simulink model "modemPSK"  (Simulink 7.1)
settings: Solver=ode45  StartTime=0.0  StopTime=0.09  RelTol=1e-3
libraries: dsparch4 x2, simulink x1, commrandsrc2 x1
settings Model: Creator=David Castro  LastModifiedBy=David Castro

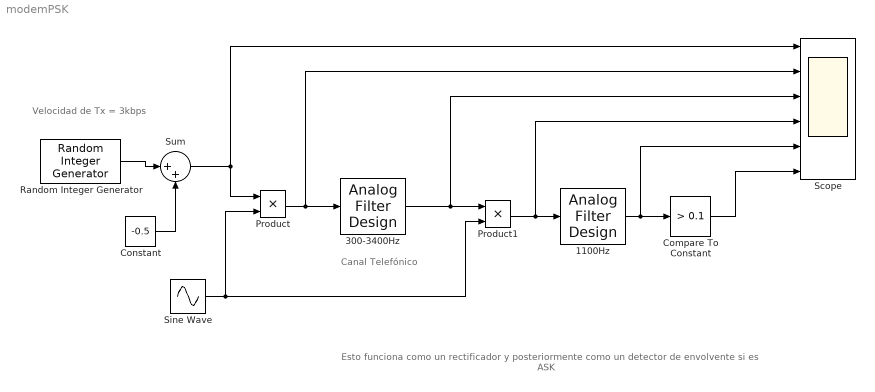
== system modemPSK ==
  note: Velocidad de Tx = 3kbps
  note: Canal Telefónico
  note: Esto funciona como un rectificador y posteriormente como un detector de envolvente si es ASK
  1100Hz : dsparch4/Analog Filter Design  method=Butterworth  filttype=Lowpass  N=2  Wlo=1200*2*pi  Whi=3400*2*pi  Rp=2  Rs=40
  300-3400Hz : dsparch4/Analog Filter Design  method=Chebyshev I  filttype=Bandpass  N=2  Wlo=300*2*pi  Whi=3400*2*pi  Rp=2  Rs=40
  Compare To Constant : simulink/Logic and Bit Operations/Compare To Constant  SystemSampleTime=-1  relop=>  const=0.1  LogicOutDataTypeMode=uint8  ZeroCross=off
  Constant : Constant  Value=-0.5  OutDataType=sfix(16)  OutScaling=2^0
  Product : Product  OutDataType=sfix(16)  OutScaling=2^0  RndMeth=Zero
  Product1 : Product  OutDataType=sfix(16)  OutScaling=2^0  RndMeth=Zero
  Random Integer Generator : commrandsrc2/Random Integer Generator  SystemSampleTime=-1  mul=2  seed=37  Ts=0.0003333333  frameBased=off  sampPerFrame=1  orient=on  outDataType=double
  Scope : Scope  NumInputPorts=6
      settings: TimeRange=0.09  YMin=-5~-5~-5~-8~-5~-5  YMax=5~5~5~8~5~5  MaxDataPoints=50000
  Sine Wave : Sin  Amplitude=2  Frequency=2000*2*pi  Samples=100  SampleTime=0.000005
  Sum : Sum  Inputs=|++  OutDataType=sfix(16)  OutScaling=2^0
  wires:
  Product/1 -> 300-3400Hz/1, Scope/2
  Sine Wave/1 -> Product/2, Product1/2
  Product1/1 -> 1100Hz/1, Scope/4
  1100Hz/1 -> Compare To Constant/1, Scope/5
  300-3400Hz/1 -> Product1/1, Scope/3
  Random Integer Generator/1 -> Sum/1
  Sum/1 -> Scope/1, Product/1
  Constant/1 -> Sum/2
  Compare To Constant/1 -> Scope/6
